simulink model "equation_1"  (R2025a)
settings: Solver=VariableStepAuto  StartTime=0.0  StopTime=10.0  RelTol=1e-3
settings Model: Creator=Johan  LastModifiedBy=Johan

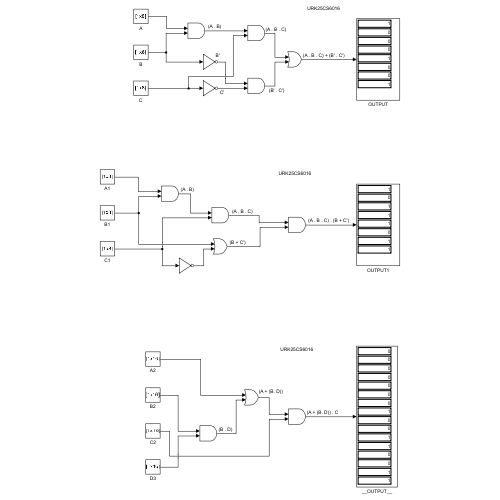
[thumbnail: Simulink's stored preview of the top-level diagram]
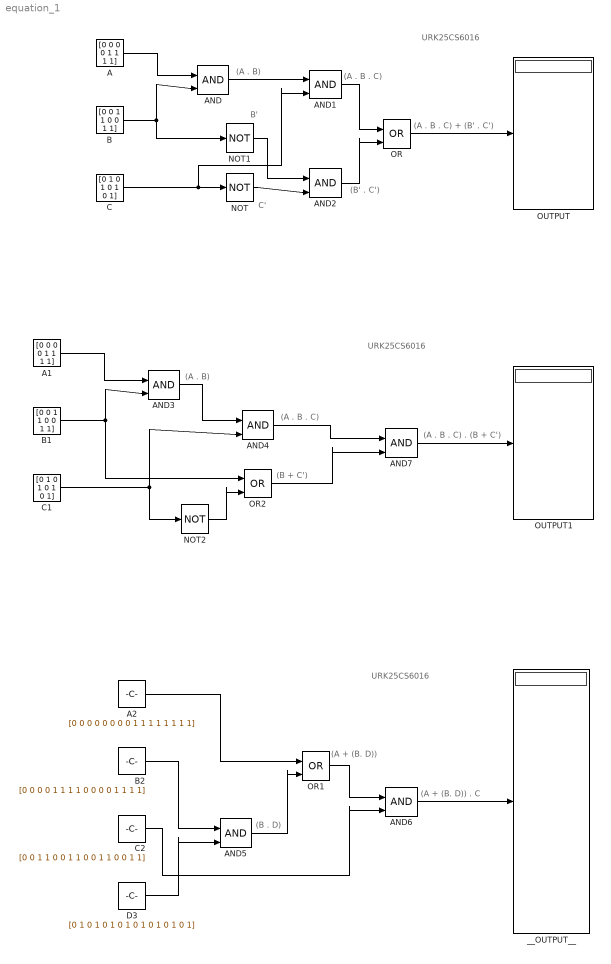
== system equation_1 ==
  note: (A . B . C) . (B + C')
  note: (B + C')
  note: (A + (B. D)) . C
  note: (A + (B. D))
  note: (B . D)
  note: URK25CS6016
  note: (A . B . C)
  note: (A . B)
  note: URK25CS6016
  note: (A . B . C) + (B' . C')
  note: (B' . C')
  note: (A . B . C)
  note: C'
  note: B'
  note: (A . B)
  note: URK25CS6016
  A : Constant  Value=[0 0 0 0 1 1 1 1]
  A1 : Constant  Value=[0 0 0 0 1 1 1 1]
  A2 : Constant  Value=[0 0 0 0 0 0 0 0 1 1 1 1 1 1 1 1]
  AND{,1..7} (8 alike) : Logic  IconShape=distinctive  AllPortsSameDT=off  OutDataTypeStr=boolean
  B : Constant  Value=[0 0 1 1 0 0 1 1]
  B1 : Constant  Value=[0 0 1 1 0 0 1 1]
  B2 : Constant  Value=[0 0 0 0 1 1 1 1 0 0 0 0 1 1 1 1]
  C : Constant  Value=[0 1 0 1 0 1 0 1]
  C1 : Constant  Value=[0 1 0 1 0 1 0 1]
  C2 : Constant  Value=[0 0 1 1 0 0 1 1 0 0 1 1 0 0 1 1]
  D3 : Constant  Value=[0 1 0 1 0 1 0 1 0 1 0 1 0 1 0 1]
  NOT : Logic  Operator=NOT  IconShape=distinctive  AllPortsSameDT=off  OutDataTypeStr=boolean
  NOT1 : Logic  Operator=NOT  IconShape=distinctive  AllPortsSameDT=off  OutDataTypeStr=boolean
  NOT2 : Logic  Operator=NOT  IconShape=distinctive  AllPortsSameDT=off  OutDataTypeStr=boolean
  OR : Logic  Operator=OR  IconShape=distinctive  AllPortsSameDT=off  OutDataTypeStr=boolean
  OR1 : Logic  Operator=OR  IconShape=distinctive  AllPortsSameDT=off  OutDataTypeStr=boolean
  OR2 : Logic  Operator=OR  IconShape=distinctive  AllPortsSameDT=off  OutDataTypeStr=boolean
  OUTPUT : Display
  OUTPUT1 : Display
  __OUTPUT__ : Display
  wires:
  A/1 -> AND/1
  B/1 -> NOT1/1, AND/2
  AND/1 -> AND1/1
  C/1 -> NOT/1, AND1/2
  NOT1/1 -> AND2/1
  NOT/1 -> AND2/2
  AND1/1 -> OR/1
  AND2/1 -> OR/2
  OR/1 -> OUTPUT/1
  A1/1 -> AND3/1
  B1/1 -> AND3/2, OR2/1
  AND3/1 -> AND4/1
  C1/1 -> NOT2/1, AND4/2
  B2/1 -> AND5/1
  D3/1 -> AND5/2
  A2/1 -> OR1/1
  AND5/1 -> OR1/2
  C2/1 -> AND6/2
  OR1/1 -> AND6/1
  AND6/1 -> __OUTPUT__/1
  NOT2/1 -> OR2/2
  AND4/1 -> AND7/1
  OR2/1 -> AND7/2
  AND7/1 -> OUTPUT1/1
